simulink model "TST_AFS_VD"  (R2016b)
settings: Solver=FixedStepDiscrete  StartTime=0.0  StopTime=simTime  FixedStep=sampleTime  RelTol=1e-3
values from neighbouring files (symbols this model uses):
  testCase = 1    [initTST_AFS_VD_001.m]    (also in initTST_AFS_VD_002.m = 2)
libraries: simulink x15, UnitTest_Lib x12
settings Model: Creator=zhengjinyan  LastModifiedBy=zhengjinyan
settings DebuggingCC: SignalRangeChecking=error
settings ConfigComp: CovEnable=on  RecordCoverage=on  CovFilter=H:\ZJY\T3_NSE_UT\build\UnitTest\AFS_VD\slcov_output\AFS_VD_covfilter.cvf  CovHTMLOptions=-sRT=0  CovHtmlReporting=on  CovSaveCumulativeToWorkspaceVar=on  CovCumulativeVarName=AFS_VD_covCumulativeData  CovCumulativeReport=on  CovShowResultsExplorer=off  CovModelRefEnable=on

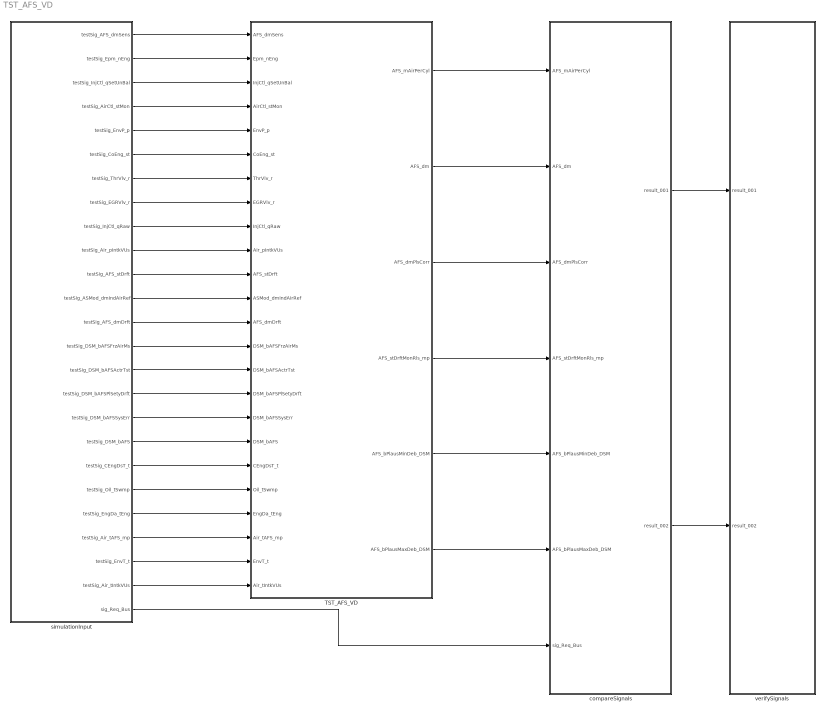
== system TST_AFS_VD ==
  TST_AFS_VD : Subsystem
  compareSignals : Subsystem
  simulationInput : Subsystem
  verifySignals : Subsystem
  wires:
  simulationInput/1(testSig_AFS_dmSens) -> TST_AFS_VD/1(AFS_dmSens)
  simulationInput/2(testSig_Epm_nEng) -> TST_AFS_VD/2(Epm_nEng)
  simulationInput/3(testSig_InjCtl_qSetUnBal) -> TST_AFS_VD/3(InjCtl_qSetUnBal)
  simulationInput/4(testSig_AirCtl_stMon) -> TST_AFS_VD/4(AirCtl_stMon)
  simulationInput/5(testSig_EnvP_p) -> TST_AFS_VD/5(EnvP_p)
  simulationInput/6(testSig_CoEng_st) -> TST_AFS_VD/6(CoEng_st)
  simulationInput/7(testSig_ThrVlv_r) -> TST_AFS_VD/7(ThrVlv_r)
  simulationInput/8(testSig_EGRVlv_r) -> TST_AFS_VD/8(EGRVlv_r)
  simulationInput/9(testSig_InjCtl_qRaw) -> TST_AFS_VD/9(InjCtl_qRaw)
  simulationInput/10(testSig_Air_pIntkVUs) -> TST_AFS_VD/10(Air_pIntkVUs)
  simulationInput/11(testSig_AFS_stDrft) -> TST_AFS_VD/11(AFS_stDrft)
  simulationInput/12(testSig_ASMod_dmIndAirRef) -> TST_AFS_VD/12(ASMod_dmIndAirRef)
  simulationInput/13(testSig_AFS_dmDrft) -> TST_AFS_VD/13(AFS_dmDrft)
  simulationInput/14(testSig_DSM_bAFSFrzAirMs) -> TST_AFS_VD/14(DSM_bAFSFrzAirMs)
  simulationInput/15(testSig_DSM_bAFSActrTst) -> TST_AFS_VD/15(DSM_bAFSActrTst)
  simulationInput/16(testSig_DSM_bAFSPlSetyDrft) -> TST_AFS_VD/16(DSM_bAFSPlSetyDrft)
  simulationInput/17(testSig_DSM_bAFSSysErr) -> TST_AFS_VD/17(DSM_bAFSSysErr)
  simulationInput/18(testSig_DSM_bAFS) -> TST_AFS_VD/18(DSM_bAFS)
  simulationInput/19(testSig_CEngDsT_t) -> TST_AFS_VD/19(CEngDsT_t)
  simulationInput/20(testSig_Oil_tSwmp) -> TST_AFS_VD/20(Oil_tSwmp)
  simulationInput/21(testSig_EngDa_tEng) -> TST_AFS_VD/21(EngDa_tEng)
  simulationInput/22(testSig_Air_tAFS_mp) -> TST_AFS_VD/22(Air_tAFS_mp)
  simulationInput/23(testSig_EnvT_t) -> TST_AFS_VD/23(EnvT_t)
  simulationInput/24(testSig_Air_tIntkVUs) -> TST_AFS_VD/24(Air_tIntkVUs)
  TST_AFS_VD/1(AFS_mAirPerCyl) -> compareSignals/1(AFS_mAirPerCyl)
  TST_AFS_VD/2(AFS_dm) -> compareSignals/2(AFS_dm)
  TST_AFS_VD/3(AFS_dmPlsCorr) -> compareSignals/3(AFS_dmPlsCorr)
  TST_AFS_VD/4(AFS_stDrftMonRls_mp) -> compareSignals/4(AFS_stDrftMonRls_mp)
  TST_AFS_VD/5(AFS_bPlausMinDeb_DSM) -> compareSignals/5(AFS_bPlausMinDeb_DSM)
  TST_AFS_VD/6(AFS_bPlausMaxDeb_DSM) -> compareSignals/6(AFS_bPlausMaxDeb_DSM)
  simulationInput/25(sig_Req_Bus) -> compareSignals/7(sig_Req_Bus)
  compareSignals/1(result_001) -> verifySignals/1(result_001)
  compareSignals/2(result_002) -> verifySignals/2(result_002)

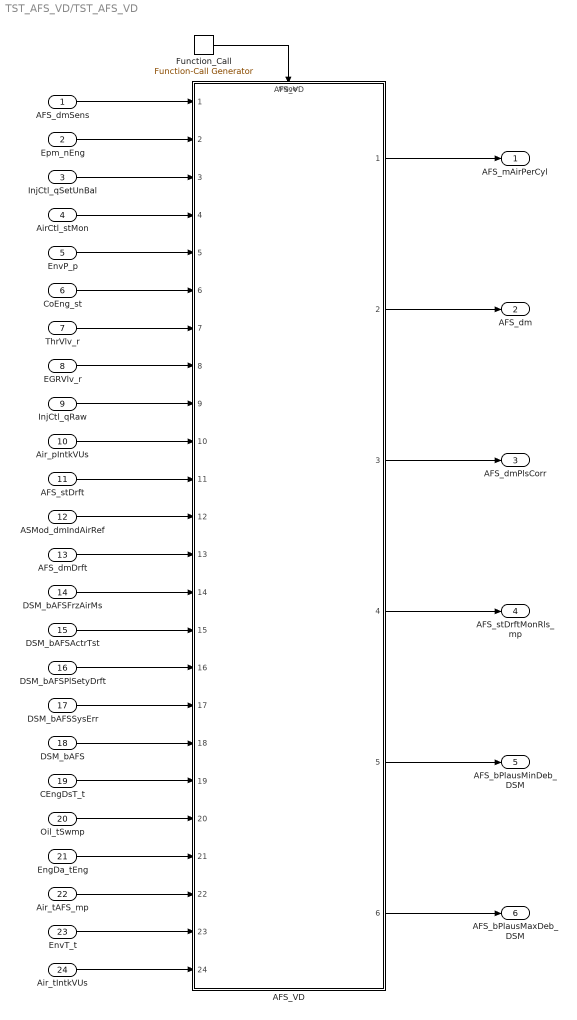
== system TST_AFS_VD/TST_AFS_VD ==
  AFS_dmSens : Inport
  Epm_nEng : Inport  Port=2
  InjCtl_qSetUnBal : Inport  Port=3
  AirCtl_stMon : Inport  Port=4
  EnvP_p : Inport  Port=5
  CoEng_st : Inport  Port=6
  ThrVlv_r : Inport  Port=7
  EGRVlv_r : Inport  Port=8
  InjCtl_qRaw : Inport  Port=9
  Air_pIntkVUs : Inport  Port=10
  AFS_stDrft : Inport  Port=11
  ASMod_dmIndAirRef : Inport  Port=12
  AFS_dmDrft : Inport  Port=13
  DSM_bAFSFrzAirMs : Inport  Port=14
  DSM_bAFSActrTst : Inport  Port=15
  DSM_bAFSPlSetyDrft : Inport  Port=16
  DSM_bAFSSysErr : Inport  Port=17
  DSM_bAFS : Inport  Port=18
  CEngDsT_t : Inport  Port=19
  Oil_tSwmp : Inport  Port=20
  EngDa_tEng : Inport  Port=21
  Air_tAFS_mp : Inport  Port=22
  EnvT_t : Inport  Port=23
  Air_tIntkVUs : Inport  Port=24
  AFS_VD : ModelReference  ModelNameDialog=AFS_VD  SimulationMode=Normal  ModelReferenceVersion=1.64  TriggerPortName=function  TriggerPortTriggerType=function-call  TriggerPortStatesWhenEnabling=held
  Function_Call : simulink/Ports & Subsystems/Function-Call Generator  sample_time=sampleTime  numberOfIterations=1
  AFS_mAirPerCyl : Outport
  AFS_dm : Outport  Port=2
  AFS_dmPlsCorr : Outport  Port=3
  AFS_stDrftMonRls_mp : Outport  Port=4
  AFS_bPlausMinDeb_DSM : Outport  Port=5
  AFS_bPlausMaxDeb_DSM : Outport  Port=6
  wires:
  Function_Call/1 -> AFS_VD/Trigger
  AFS_dmSens/1 -> AFS_VD/1
  Epm_nEng/1 -> AFS_VD/2
  InjCtl_qSetUnBal/1 -> AFS_VD/3
  AirCtl_stMon/1 -> AFS_VD/4
  EnvP_p/1 -> AFS_VD/5
  CoEng_st/1 -> AFS_VD/6
  ThrVlv_r/1 -> AFS_VD/7
  EGRVlv_r/1 -> AFS_VD/8
  InjCtl_qRaw/1 -> AFS_VD/9
  Air_pIntkVUs/1 -> AFS_VD/10
  AFS_stDrft/1 -> AFS_VD/11
  ASMod_dmIndAirRef/1 -> AFS_VD/12
  AFS_dmDrft/1 -> AFS_VD/13
  DSM_bAFSFrzAirMs/1 -> AFS_VD/14
  DSM_bAFSActrTst/1 -> AFS_VD/15
  DSM_bAFSPlSetyDrft/1 -> AFS_VD/16
  DSM_bAFSSysErr/1 -> AFS_VD/17
  DSM_bAFS/1 -> AFS_VD/18
  CEngDsT_t/1 -> AFS_VD/19
  Oil_tSwmp/1 -> AFS_VD/20
  EngDa_tEng/1 -> AFS_VD/21
  Air_tAFS_mp/1 -> AFS_VD/22
  EnvT_t/1 -> AFS_VD/23
  Air_tIntkVUs/1 -> AFS_VD/24
  AFS_VD/1 -> AFS_mAirPerCyl/1
  AFS_VD/2 -> AFS_dm/1
  AFS_VD/3 -> AFS_dmPlsCorr/1
  AFS_VD/4 -> AFS_stDrftMonRls_mp/1
  AFS_VD/5 -> AFS_bPlausMinDeb_DSM/1
  AFS_VD/6 -> AFS_bPlausMaxDeb_DSM/1

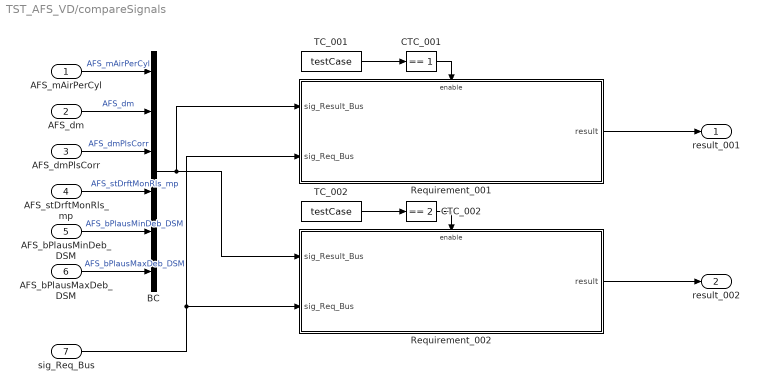
== system TST_AFS_VD/compareSignals ==
  AFS_mAirPerCyl : Inport
  AFS_dm : Inport  Port=2
  AFS_dmPlsCorr : Inport  Port=3
  AFS_stDrftMonRls_mp : Inport  Port=4
  AFS_bPlausMinDeb_DSM : Inport  Port=5
  AFS_bPlausMaxDeb_DSM : Inport  Port=6
  sig_Req_Bus : Inport  Port=7
  BC : BusCreator  Inputs=6
  CTC_001 : simulink/Logic and Bit Operations/Compare To Constant  relop===  const=1  OutDataTypeStr=boolean
  CTC_002 : simulink/Logic and Bit Operations/Compare To Constant  relop===  const=2  OutDataTypeStr=boolean
  Requirement_001 : Subsystem
  Requirement_002 : Subsystem
  TC_001 : Constant  Value=testCase
  TC_002 : Constant  Value=testCase
  result_001 : Outport
  result_002 : Outport  Port=2
  wires:
  AFS_mAirPerCyl/1 -> BC/1  "AFS_mAirPerCyl"
  AFS_dm/1 -> BC/2  "AFS_dm"
  AFS_dmPlsCorr/1 -> BC/3  "AFS_dmPlsCorr"
  AFS_stDrftMonRls_mp/1 -> BC/4  "AFS_stDrftMonRls_mp"
  AFS_bPlausMinDeb_DSM/1 -> BC/5  "AFS_bPlausMinDeb_DSM"
  AFS_bPlausMaxDeb_DSM/1 -> BC/6  "AFS_bPlausMaxDeb_DSM"
  TC_001/1 -> CTC_001/1
  CTC_001/1 -> Requirement_001/Enable
  sig_Req_Bus/1 -> Requirement_001/2(sig_Req_Bus), Requirement_002/2(sig_Req_Bus)
  BC/1 -> Requirement_001/1(sig_Result_Bus), Requirement_002/1(sig_Result_Bus)
  Requirement_001/1(result) -> result_001/1
  TC_002/1 -> CTC_002/1
  CTC_002/1 -> Requirement_002/Enable
  Requirement_002/1(result) -> result_002/1

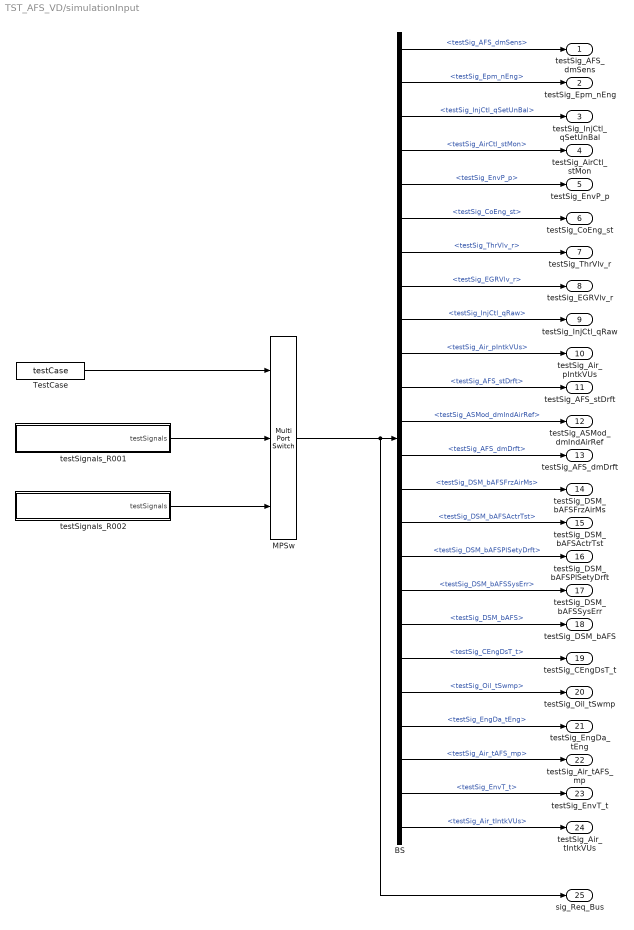
== system TST_AFS_VD/simulationInput ==
  BS : BusSelector  OutputSignals=testSig_AFS_dmSens,testSig_Epm_nEng,testSig_InjCtl_qSetUnBal,testSig_AirCtl_stMon,testSig_EnvP_p,testSig_CoEng_st,testSig_ThrVlv_r,testSig_EGRVlv_r,testSig_InjCtl_qRaw,testSig_Air_pIntkVUs,testSig_AFS_stDrft,testSig_ASMod_dmIndAirRef,testSig_AFS_dmDrft,testSig_DSM_bAFSFrzAirMs,testSig_DSM_bAFSActrTst,testSig_DSM_bAFSPlSetyDrft,testSig_DSM_bAFSSysErr,testSig_DSM_bAFS,testSig_CEngDsT_t,testSig_Oil_tSwmp,testSig_EngDa_tEng,testSig_Air_tAFS_mp,testSig_EnvT_t,testSig_Air_tIntkVUs
  MPSw : MultiPortSwitch  Inputs=2  SaturateOnIntegerOverflow=on  InputSameDT=on
  TestCase : Constant  Value=testCase
  testSignals_R001 : Subsystem
  testSignals_R002 : Subsystem
  testSig_AFS_dmSens : Outport
  testSig_Epm_nEng : Outport  Port=2
  testSig_InjCtl_qSetUnBal : Outport  Port=3
  testSig_AirCtl_stMon : Outport  Port=4
  testSig_EnvP_p : Outport  Port=5
  testSig_CoEng_st : Outport  Port=6
  testSig_ThrVlv_r : Outport  Port=7
  testSig_EGRVlv_r : Outport  Port=8
  testSig_InjCtl_qRaw : Outport  Port=9
  testSig_Air_pIntkVUs : Outport  Port=10
  testSig_AFS_stDrft : Outport  Port=11
  testSig_ASMod_dmIndAirRef : Outport  Port=12
  testSig_AFS_dmDrft : Outport  Port=13
  testSig_DSM_bAFSFrzAirMs : Outport  Port=14
  testSig_DSM_bAFSActrTst : Outport  Port=15
  testSig_DSM_bAFSPlSetyDrft : Outport  Port=16
  testSig_DSM_bAFSSysErr : Outport  Port=17
  testSig_DSM_bAFS : Outport  Port=18
  testSig_CEngDsT_t : Outport  Port=19
  testSig_Oil_tSwmp : Outport  Port=20
  testSig_EngDa_tEng : Outport  Port=21
  testSig_Air_tAFS_mp : Outport  Port=22
  testSig_EnvT_t : Outport  Port=23
  testSig_Air_tIntkVUs : Outport  Port=24
  sig_Req_Bus : Outport  Port=25
  wires:
  BS/1 -> testSig_AFS_dmSens/1  "<testSig_AFS_dmSens>"
  BS/2 -> testSig_Epm_nEng/1  "<testSig_Epm_nEng>"
  BS/3 -> testSig_InjCtl_qSetUnBal/1  "<testSig_InjCtl_qSetUnBal>"
  BS/4 -> testSig_AirCtl_stMon/1  "<testSig_AirCtl_stMon>"
  BS/5 -> testSig_EnvP_p/1  "<testSig_EnvP_p>"
  BS/6 -> testSig_CoEng_st/1  "<testSig_CoEng_st>"
  BS/7 -> testSig_ThrVlv_r/1  "<testSig_ThrVlv_r>"
  BS/8 -> testSig_EGRVlv_r/1  "<testSig_EGRVlv_r>"
  BS/9 -> testSig_InjCtl_qRaw/1  "<testSig_InjCtl_qRaw>"
  BS/10 -> testSig_Air_pIntkVUs/1  "<testSig_Air_pIntkVUs>"
  BS/11 -> testSig_AFS_stDrft/1  "<testSig_AFS_stDrft>"
  BS/12 -> testSig_ASMod_dmIndAirRef/1  "<testSig_ASMod_dmIndAirRef>"
  BS/13 -> testSig_AFS_dmDrft/1  "<testSig_AFS_dmDrft>"
  BS/14 -> testSig_DSM_bAFSFrzAirMs/1  "<testSig_DSM_bAFSFrzAirMs>"
  BS/15 -> testSig_DSM_bAFSActrTst/1  "<testSig_DSM_bAFSActrTst>"
  BS/16 -> testSig_DSM_bAFSPlSetyDrft/1  "<testSig_DSM_bAFSPlSetyDrft>"
  BS/17 -> testSig_DSM_bAFSSysErr/1  "<testSig_DSM_bAFSSysErr>"
  BS/18 -> testSig_DSM_bAFS/1  "<testSig_DSM_bAFS>"
  BS/19 -> testSig_CEngDsT_t/1  "<testSig_CEngDsT_t>"
  BS/20 -> testSig_Oil_tSwmp/1  "<testSig_Oil_tSwmp>"
  BS/21 -> testSig_EngDa_tEng/1  "<testSig_EngDa_tEng>"
  BS/22 -> testSig_Air_tAFS_mp/1  "<testSig_Air_tAFS_mp>"
  BS/23 -> testSig_EnvT_t/1  "<testSig_EnvT_t>"
  BS/24 -> testSig_Air_tIntkVUs/1  "<testSig_Air_tIntkVUs>"
  MPSw/1 -> BS/1, sig_Req_Bus/1
  TestCase/1 -> MPSw/1
  testSignals_R001/1(testSignals) -> MPSw/2
  testSignals_R002/1(testSignals) -> MPSw/3

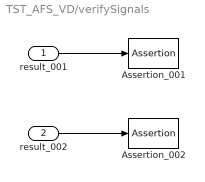
== system TST_AFS_VD/verifySignals ==
  result_001 : Inport
  result_002 : Inport  Port=2
  Assertion_001 : Assertion  Enabled=off
  Assertion_002 : Assertion  Enabled=off
  wires:
  result_001/1 -> Assertion_001/1
  result_002/1 -> Assertion_002/1

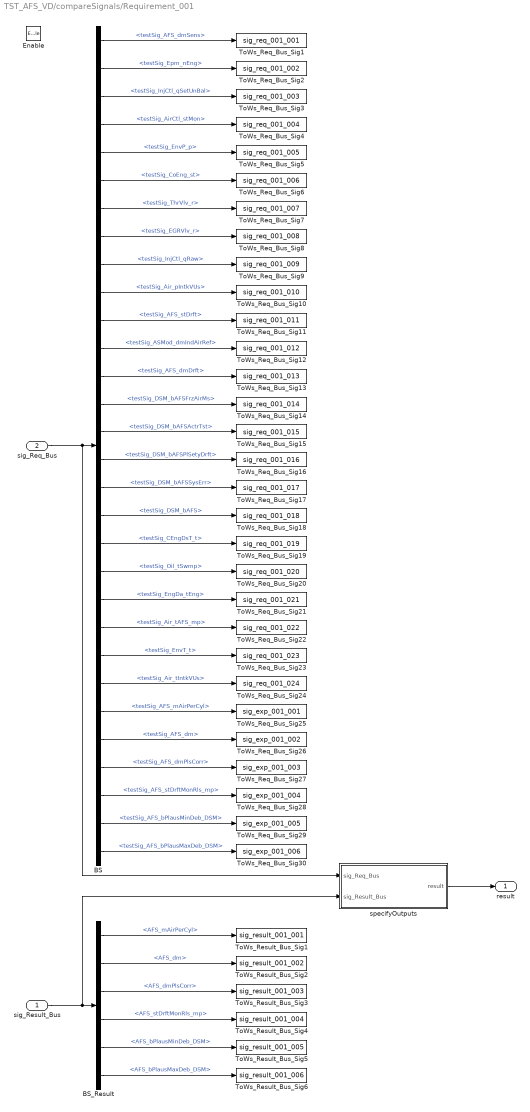
== system TST_AFS_VD/compareSignals/Requirement_001 ==
  sig_Result_Bus : Inport
  sig_Req_Bus : Inport  Port=2
  Enable : EnablePort
  BS : BusSelector  OutputSignals=testSig_AFS_dmSens,testSig_Epm_nEng,testSig_InjCtl_qSetUnBal,testSig_AirCtl_stMon,testSig_EnvP_p,testSig_CoEng_st,testSig_ThrVlv_r,testSig_EGRVlv_r,testSig_InjCtl_qRaw,testSig_Air_pIntkVUs,testSig_AFS_stDrft,testSig_ASMod_dmIndAirRef,testSig_AFS_dmDrft,testSig_DSM_bAFSFrzAirMs,testSig_DSM_bAFSActrTst,testSig_DSM_bAFSPlSetyDrft,testSig_DSM_bAFSSysErr,testSig_DSM_bAFS,testSig_CEngDsT_t,testSig_Oil_tSwmp,testSig_EngDa_tEng,testSig_Air_tAFS_mp,testSig_EnvT_t,testSig_Air_tIntkVUs,testSig_AFS_mAirPerCyl,testSig_AFS_dm,testSig_AFS_dmPlsCorr,testSig_AFS_stDrftMonRls_mp,testSig_AFS_bPlausMinDeb_DSM,testSig_AFS_bPlausMaxDeb_DSM
  BS_Result : BusSelector  OutputSignals=AFS_mAirPerCyl,AFS_dm,AFS_dmPlsCorr,AFS_stDrftMonRls_mp,AFS_bPlausMinDeb_DSM,AFS_bPlausMaxDeb_DSM
  ToWs_Req_Bus_Sig1 : ToWorkspace  VariableName=sig_req_001_001  SaveFormat=Structure With Time
  ToWs_Req_Bus_Sig10 : ToWorkspace  VariableName=sig_req_001_010  SaveFormat=Structure With Time
  ToWs_Req_Bus_Sig11 : ToWorkspace  VariableName=sig_req_001_011  SaveFormat=Structure With Time
  ToWs_Req_Bus_Sig12 : ToWorkspace  VariableName=sig_req_001_012  SaveFormat=Structure With Time
  ToWs_Req_Bus_Sig13 : ToWorkspace  VariableName=sig_req_001_013  SaveFormat=Structure With Time
  ToWs_Req_Bus_Sig14 : ToWorkspace  VariableName=sig_req_001_014  SaveFormat=Structure With Time
  ToWs_Req_Bus_Sig15 : ToWorkspace  VariableName=sig_req_001_015  SaveFormat=Structure With Time
  ToWs_Req_Bus_Sig16 : ToWorkspace  VariableName=sig_req_001_016  SaveFormat=Structure With Time
  ToWs_Req_Bus_Sig17 : ToWorkspace  VariableName=sig_req_001_017  SaveFormat=Structure With Time
  ToWs_Req_Bus_Sig18 : ToWorkspace  VariableName=sig_req_001_018  SaveFormat=Structure With Time
  ToWs_Req_Bus_Sig19 : ToWorkspace  VariableName=sig_req_001_019  SaveFormat=Structure With Time
  ToWs_Req_Bus_Sig2 : ToWorkspace  VariableName=sig_req_001_002  SaveFormat=Structure With Time
  ToWs_Req_Bus_Sig20 : ToWorkspace  VariableName=sig_req_001_020  SaveFormat=Structure With Time
  ToWs_Req_Bus_Sig21 : ToWorkspace  VariableName=sig_req_001_021  SaveFormat=Structure With Time
  ToWs_Req_Bus_Sig22 : ToWorkspace  VariableName=sig_req_001_022  SaveFormat=Structure With Time
  ToWs_Req_Bus_Sig23 : ToWorkspace  VariableName=sig_req_001_023  SaveFormat=Structure With Time
  ToWs_Req_Bus_Sig24 : ToWorkspace  VariableName=sig_req_001_024  SaveFormat=Structure With Time
  ToWs_Req_Bus_Sig25 : ToWorkspace  VariableName=sig_exp_001_001  SaveFormat=Structure With Time
  ToWs_Req_Bus_Sig26 : ToWorkspace  VariableName=sig_exp_001_002  SaveFormat=Structure With Time
  ToWs_Req_Bus_Sig27 : ToWorkspace  VariableName=sig_exp_001_003  SaveFormat=Structure With Time
  ToWs_Req_Bus_Sig28 : ToWorkspace  VariableName=sig_exp_001_004  SaveFormat=Structure With Time
  ToWs_Req_Bus_Sig29 : ToWorkspace  VariableName=sig_exp_001_005  SaveFormat=Structure With Time
  ToWs_Req_Bus_Sig3 : ToWorkspace  VariableName=sig_req_001_003  SaveFormat=Structure With Time
  ToWs_Req_Bus_Sig30 : ToWorkspace  VariableName=sig_exp_001_006  SaveFormat=Structure With Time
  ToWs_Req_Bus_Sig4 : ToWorkspace  VariableName=sig_req_001_004  SaveFormat=Structure With Time
  ToWs_Req_Bus_Sig5 : ToWorkspace  VariableName=sig_req_001_005  SaveFormat=Structure With Time
  ToWs_Req_Bus_Sig6 : ToWorkspace  VariableName=sig_req_001_006  SaveFormat=Structure With Time
  ToWs_Req_Bus_Sig7 : ToWorkspace  VariableName=sig_req_001_007  SaveFormat=Structure With Time
  ToWs_Req_Bus_Sig8 : ToWorkspace  VariableName=sig_req_001_008  SaveFormat=Structure With Time
  ToWs_Req_Bus_Sig9 : ToWorkspace  VariableName=sig_req_001_009  SaveFormat=Structure With Time
  ToWs_Result_Bus_Sig1 : ToWorkspace  VariableName=sig_result_001_001  SaveFormat=Structure With Time
  ToWs_Result_Bus_Sig2 : ToWorkspace  VariableName=sig_result_001_002  SaveFormat=Structure With Time
  ToWs_Result_Bus_Sig3 : ToWorkspace  VariableName=sig_result_001_003  SaveFormat=Structure With Time
  ToWs_Result_Bus_Sig4 : ToWorkspace  VariableName=sig_result_001_004  SaveFormat=Structure With Time
  ToWs_Result_Bus_Sig5 : ToWorkspace  VariableName=sig_result_001_005  SaveFormat=Structure With Time
  ToWs_Result_Bus_Sig6 : ToWorkspace  VariableName=sig_result_001_006  SaveFormat=Structure With Time
  specifyOutputs : Subsystem
  result : Outport
  wires:
  sig_Req_Bus/1 -> BS/1, specifyOutputs/1(sig_Req_Bus)
  BS/1 -> ToWs_Req_Bus_Sig1/1  "<testSig_AFS_dmSens>"
  BS/2 -> ToWs_Req_Bus_Sig2/1  "<testSig_Epm_nEng>"
  BS/3 -> ToWs_Req_Bus_Sig3/1  "<testSig_InjCtl_qSetUnBal>"
  BS/4 -> ToWs_Req_Bus_Sig4/1  "<testSig_AirCtl_stMon>"
  BS/5 -> ToWs_Req_Bus_Sig5/1  "<testSig_EnvP_p>"
  BS/6 -> ToWs_Req_Bus_Sig6/1  "<testSig_CoEng_st>"
  BS/7 -> ToWs_Req_Bus_Sig7/1  "<testSig_ThrVlv_r>"
  BS/8 -> ToWs_Req_Bus_Sig8/1  "<testSig_EGRVlv_r>"
  BS/9 -> ToWs_Req_Bus_Sig9/1  "<testSig_InjCtl_qRaw>"
  BS/10 -> ToWs_Req_Bus_Sig10/1  "<testSig_Air_pIntkVUs>"
  BS/11 -> ToWs_Req_Bus_Sig11/1  "<testSig_AFS_stDrft>"
  BS/12 -> ToWs_Req_Bus_Sig12/1  "<testSig_ASMod_dmIndAirRef>"
  BS/13 -> ToWs_Req_Bus_Sig13/1  "<testSig_AFS_dmDrft>"
  BS/14 -> ToWs_Req_Bus_Sig14/1  "<testSig_DSM_bAFSFrzAirMs>"
  BS/15 -> ToWs_Req_Bus_Sig15/1  "<testSig_DSM_bAFSActrTst>"
  BS/16 -> ToWs_Req_Bus_Sig16/1  "<testSig_DSM_bAFSPlSetyDrft>"
  BS/17 -> ToWs_Req_Bus_Sig17/1  "<testSig_DSM_bAFSSysErr>"
  BS/18 -> ToWs_Req_Bus_Sig18/1  "<testSig_DSM_bAFS>"
  BS/19 -> ToWs_Req_Bus_Sig19/1  "<testSig_CEngDsT_t>"
  BS/20 -> ToWs_Req_Bus_Sig20/1  "<testSig_Oil_tSwmp>"
  BS/21 -> ToWs_Req_Bus_Sig21/1  "<testSig_EngDa_tEng>"
  BS/22 -> ToWs_Req_Bus_Sig22/1  "<testSig_Air_tAFS_mp>"
  BS/23 -> ToWs_Req_Bus_Sig23/1  "<testSig_EnvT_t>"
  BS/24 -> ToWs_Req_Bus_Sig24/1  "<testSig_Air_tIntkVUs>"
  BS/25 -> ToWs_Req_Bus_Sig25/1  "<testSig_AFS_mAirPerCyl>"
  BS/26 -> ToWs_Req_Bus_Sig26/1  "<testSig_AFS_dm>"
  BS/27 -> ToWs_Req_Bus_Sig27/1  "<testSig_AFS_dmPlsCorr>"
  BS/28 -> ToWs_Req_Bus_Sig28/1  "<testSig_AFS_stDrftMonRls_mp>"
  BS/29 -> ToWs_Req_Bus_Sig29/1  "<testSig_AFS_bPlausMinDeb_DSM>"
  BS/30 -> ToWs_Req_Bus_Sig30/1  "<testSig_AFS_bPlausMaxDeb_DSM>"
  sig_Result_Bus/1 -> BS_Result/1, specifyOutputs/2(sig_Result_Bus)
  BS_Result/1 -> ToWs_Result_Bus_Sig1/1  "<AFS_mAirPerCyl>"
  BS_Result/2 -> ToWs_Result_Bus_Sig2/1  "<AFS_dm>"
  BS_Result/3 -> ToWs_Result_Bus_Sig3/1  "<AFS_dmPlsCorr>"
  BS_Result/4 -> ToWs_Result_Bus_Sig4/1  "<AFS_stDrftMonRls_mp>"
  BS_Result/5 -> ToWs_Result_Bus_Sig5/1  "<AFS_bPlausMinDeb_DSM>"
  BS_Result/6 -> ToWs_Result_Bus_Sig6/1  "<AFS_bPlausMaxDeb_DSM>"
  specifyOutputs/1(result) -> result/1

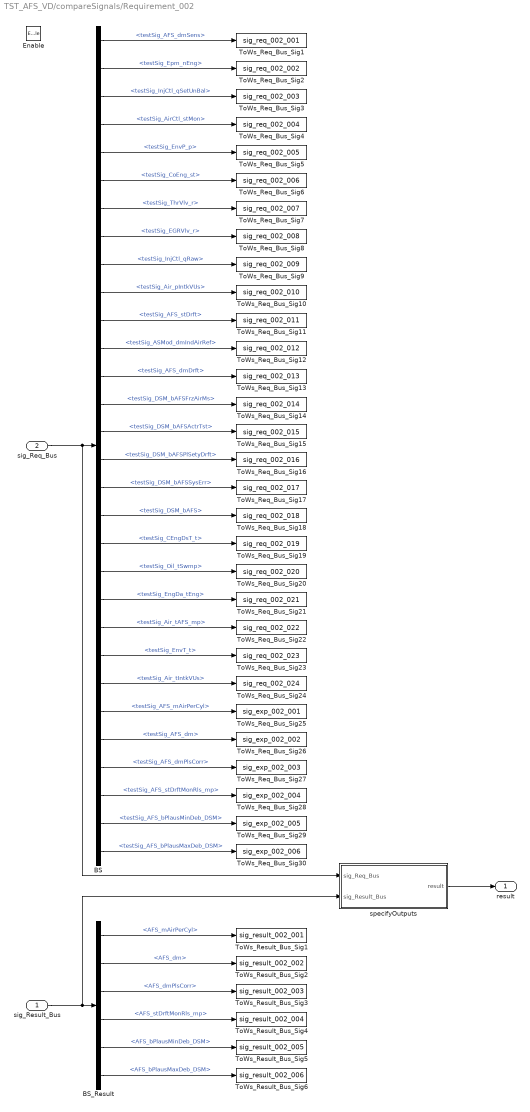
== system TST_AFS_VD/compareSignals/Requirement_002 ==
  sig_Result_Bus : Inport
  sig_Req_Bus : Inport  Port=2
  Enable : EnablePort
  BS : BusSelector  OutputSignals=testSig_AFS_dmSens,testSig_Epm_nEng,testSig_InjCtl_qSetUnBal,testSig_AirCtl_stMon,testSig_EnvP_p,testSig_CoEng_st,testSig_ThrVlv_r,testSig_EGRVlv_r,testSig_InjCtl_qRaw,testSig_Air_pIntkVUs,testSig_AFS_stDrft,testSig_ASMod_dmIndAirRef,testSig_AFS_dmDrft,testSig_DSM_bAFSFrzAirMs,testSig_DSM_bAFSActrTst,testSig_DSM_bAFSPlSetyDrft,testSig_DSM_bAFSSysErr,testSig_DSM_bAFS,testSig_CEngDsT_t,testSig_Oil_tSwmp,testSig_EngDa_tEng,testSig_Air_tAFS_mp,testSig_EnvT_t,testSig_Air_tIntkVUs,testSig_AFS_mAirPerCyl,testSig_AFS_dm,testSig_AFS_dmPlsCorr,testSig_AFS_stDrftMonRls_mp,testSig_AFS_bPlausMinDeb_DSM,testSig_AFS_bPlausMaxDeb_DSM
  BS_Result : BusSelector  OutputSignals=AFS_mAirPerCyl,AFS_dm,AFS_dmPlsCorr,AFS_stDrftMonRls_mp,AFS_bPlausMinDeb_DSM,AFS_bPlausMaxDeb_DSM
  ToWs_Req_Bus_Sig1 : ToWorkspace  VariableName=sig_req_002_001  SaveFormat=Structure With Time
  ToWs_Req_Bus_Sig10 : ToWorkspace  VariableName=sig_req_002_010  SaveFormat=Structure With Time
  ToWs_Req_Bus_Sig11 : ToWorkspace  VariableName=sig_req_002_011  SaveFormat=Structure With Time
  ToWs_Req_Bus_Sig12 : ToWorkspace  VariableName=sig_req_002_012  SaveFormat=Structure With Time
  ToWs_Req_Bus_Sig13 : ToWorkspace  VariableName=sig_req_002_013  SaveFormat=Structure With Time
  ToWs_Req_Bus_Sig14 : ToWorkspace  VariableName=sig_req_002_014  SaveFormat=Structure With Time
  ToWs_Req_Bus_Sig15 : ToWorkspace  VariableName=sig_req_002_015  SaveFormat=Structure With Time
  ToWs_Req_Bus_Sig16 : ToWorkspace  VariableName=sig_req_002_016  SaveFormat=Structure With Time
  ToWs_Req_Bus_Sig17 : ToWorkspace  VariableName=sig_req_002_017  SaveFormat=Structure With Time
  ToWs_Req_Bus_Sig18 : ToWorkspace  VariableName=sig_req_002_018  SaveFormat=Structure With Time
  ToWs_Req_Bus_Sig19 : ToWorkspace  VariableName=sig_req_002_019  SaveFormat=Structure With Time
  ToWs_Req_Bus_Sig2 : ToWorkspace  VariableName=sig_req_002_002  SaveFormat=Structure With Time
  ToWs_Req_Bus_Sig20 : ToWorkspace  VariableName=sig_req_002_020  SaveFormat=Structure With Time
  ToWs_Req_Bus_Sig21 : ToWorkspace  VariableName=sig_req_002_021  SaveFormat=Structure With Time
  ToWs_Req_Bus_Sig22 : ToWorkspace  VariableName=sig_req_002_022  SaveFormat=Structure With Time
  ToWs_Req_Bus_Sig23 : ToWorkspace  VariableName=sig_req_002_023  SaveFormat=Structure With Time
  ToWs_Req_Bus_Sig24 : ToWorkspace  VariableName=sig_req_002_024  SaveFormat=Structure With Time
  ToWs_Req_Bus_Sig25 : ToWorkspace  VariableName=sig_exp_002_001  SaveFormat=Structure With Time
  ToWs_Req_Bus_Sig26 : ToWorkspace  VariableName=sig_exp_002_002  SaveFormat=Structure With Time
  ToWs_Req_Bus_Sig27 : ToWorkspace  VariableName=sig_exp_002_003  SaveFormat=Structure With Time
  ToWs_Req_Bus_Sig28 : ToWorkspace  VariableName=sig_exp_002_004  SaveFormat=Structure With Time
  ToWs_Req_Bus_Sig29 : ToWorkspace  VariableName=sig_exp_002_005  SaveFormat=Structure With Time
  ToWs_Req_Bus_Sig3 : ToWorkspace  VariableName=sig_req_002_003  SaveFormat=Structure With Time
  ToWs_Req_Bus_Sig30 : ToWorkspace  VariableName=sig_exp_002_006  SaveFormat=Structure With Time
  ToWs_Req_Bus_Sig4 : ToWorkspace  VariableName=sig_req_002_004  SaveFormat=Structure With Time
  ToWs_Req_Bus_Sig5 : ToWorkspace  VariableName=sig_req_002_005  SaveFormat=Structure With Time
  ToWs_Req_Bus_Sig6 : ToWorkspace  VariableName=sig_req_002_006  SaveFormat=Structure With Time
  ToWs_Req_Bus_Sig7 : ToWorkspace  VariableName=sig_req_002_007  SaveFormat=Structure With Time
  ToWs_Req_Bus_Sig8 : ToWorkspace  VariableName=sig_req_002_008  SaveFormat=Structure With Time
  ToWs_Req_Bus_Sig9 : ToWorkspace  VariableName=sig_req_002_009  SaveFormat=Structure With Time
  ToWs_Result_Bus_Sig1 : ToWorkspace  VariableName=sig_result_002_001  SaveFormat=Structure With Time
  ToWs_Result_Bus_Sig2 : ToWorkspace  VariableName=sig_result_002_002  SaveFormat=Structure With Time
  ToWs_Result_Bus_Sig3 : ToWorkspace  VariableName=sig_result_002_003  SaveFormat=Structure With Time
  ToWs_Result_Bus_Sig4 : ToWorkspace  VariableName=sig_result_002_004  SaveFormat=Structure With Time
  ToWs_Result_Bus_Sig5 : ToWorkspace  VariableName=sig_result_002_005  SaveFormat=Structure With Time
  ToWs_Result_Bus_Sig6 : ToWorkspace  VariableName=sig_result_002_006  SaveFormat=Structure With Time
  specifyOutputs : Subsystem
  result : Outport
  wires:
  sig_Req_Bus/1 -> BS/1, specifyOutputs/1(sig_Req_Bus)
  BS/1 -> ToWs_Req_Bus_Sig1/1  "<testSig_AFS_dmSens>"
  BS/2 -> ToWs_Req_Bus_Sig2/1  "<testSig_Epm_nEng>"
  BS/3 -> ToWs_Req_Bus_Sig3/1  "<testSig_InjCtl_qSetUnBal>"
  BS/4 -> ToWs_Req_Bus_Sig4/1  "<testSig_AirCtl_stMon>"
  BS/5 -> ToWs_Req_Bus_Sig5/1  "<testSig_EnvP_p>"
  BS/6 -> ToWs_Req_Bus_Sig6/1  "<testSig_CoEng_st>"
  BS/7 -> ToWs_Req_Bus_Sig7/1  "<testSig_ThrVlv_r>"
  BS/8 -> ToWs_Req_Bus_Sig8/1  "<testSig_EGRVlv_r>"
  BS/9 -> ToWs_Req_Bus_Sig9/1  "<testSig_InjCtl_qRaw>"
  BS/10 -> ToWs_Req_Bus_Sig10/1  "<testSig_Air_pIntkVUs>"
  BS/11 -> ToWs_Req_Bus_Sig11/1  "<testSig_AFS_stDrft>"
  BS/12 -> ToWs_Req_Bus_Sig12/1  "<testSig_ASMod_dmIndAirRef>"
  BS/13 -> ToWs_Req_Bus_Sig13/1  "<testSig_AFS_dmDrft>"
  BS/14 -> ToWs_Req_Bus_Sig14/1  "<testSig_DSM_bAFSFrzAirMs>"
  BS/15 -> ToWs_Req_Bus_Sig15/1  "<testSig_DSM_bAFSActrTst>"
  BS/16 -> ToWs_Req_Bus_Sig16/1  "<testSig_DSM_bAFSPlSetyDrft>"
  BS/17 -> ToWs_Req_Bus_Sig17/1  "<testSig_DSM_bAFSSysErr>"
  BS/18 -> ToWs_Req_Bus_Sig18/1  "<testSig_DSM_bAFS>"
  BS/19 -> ToWs_Req_Bus_Sig19/1  "<testSig_CEngDsT_t>"
  BS/20 -> ToWs_Req_Bus_Sig20/1  "<testSig_Oil_tSwmp>"
  BS/21 -> ToWs_Req_Bus_Sig21/1  "<testSig_EngDa_tEng>"
  BS/22 -> ToWs_Req_Bus_Sig22/1  "<testSig_Air_tAFS_mp>"
  BS/23 -> ToWs_Req_Bus_Sig23/1  "<testSig_EnvT_t>"
  BS/24 -> ToWs_Req_Bus_Sig24/1  "<testSig_Air_tIntkVUs>"
  BS/25 -> ToWs_Req_Bus_Sig25/1  "<testSig_AFS_mAirPerCyl>"
  BS/26 -> ToWs_Req_Bus_Sig26/1  "<testSig_AFS_dm>"
  BS/27 -> ToWs_Req_Bus_Sig27/1  "<testSig_AFS_dmPlsCorr>"
  BS/28 -> ToWs_Req_Bus_Sig28/1  "<testSig_AFS_stDrftMonRls_mp>"
  BS/29 -> ToWs_Req_Bus_Sig29/1  "<testSig_AFS_bPlausMinDeb_DSM>"
  BS/30 -> ToWs_Req_Bus_Sig30/1  "<testSig_AFS_bPlausMaxDeb_DSM>"
  sig_Result_Bus/1 -> BS_Result/1, specifyOutputs/2(sig_Result_Bus)
  BS_Result/1 -> ToWs_Result_Bus_Sig1/1  "<AFS_mAirPerCyl>"
  BS_Result/2 -> ToWs_Result_Bus_Sig2/1  "<AFS_dm>"
  BS_Result/3 -> ToWs_Result_Bus_Sig3/1  "<AFS_dmPlsCorr>"
  BS_Result/4 -> ToWs_Result_Bus_Sig4/1  "<AFS_stDrftMonRls_mp>"
  BS_Result/5 -> ToWs_Result_Bus_Sig5/1  "<AFS_bPlausMinDeb_DSM>"
  BS_Result/6 -> ToWs_Result_Bus_Sig6/1  "<AFS_bPlausMaxDeb_DSM>"
  specifyOutputs/1(result) -> result/1

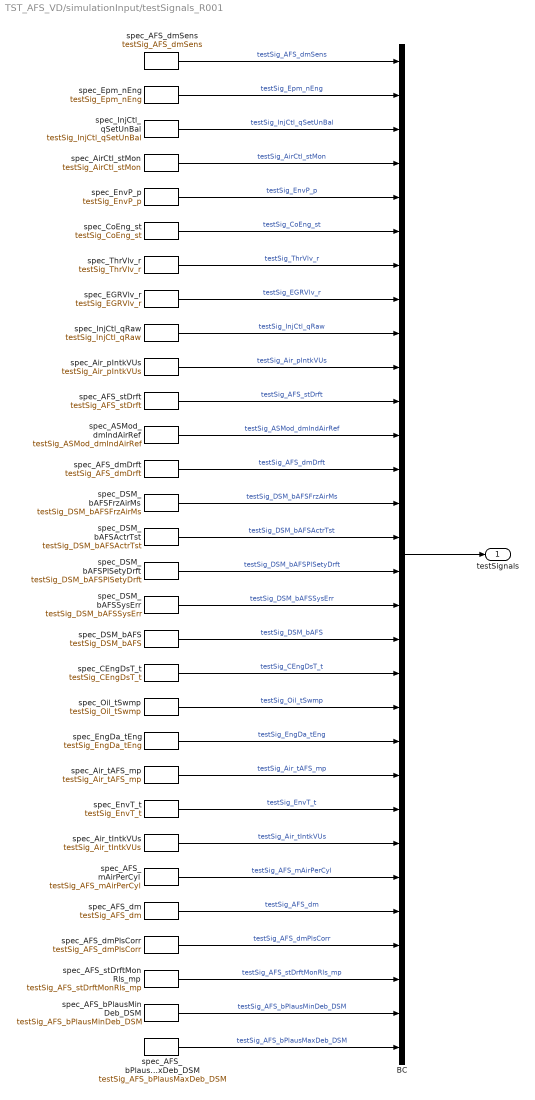
== system TST_AFS_VD/simulationInput/testSignals_R001 ==
  BC : BusCreator  Inputs=30
  spec_AFS_bPlausMaxDeb_DSM : FromWorkspace  VariableName=testSig_AFS_bPlausMaxDeb_DSM  Interpolate=off  OutputAfterFinalValue=Holding final value
  spec_AFS_bPlausMinDeb_DSM : FromWorkspace  VariableName=testSig_AFS_bPlausMinDeb_DSM  Interpolate=off  OutputAfterFinalValue=Holding final value
  spec_AFS_dm : FromWorkspace  VariableName=testSig_AFS_dm  Interpolate=off  OutputAfterFinalValue=Holding final value
  spec_AFS_dmDrft : FromWorkspace  VariableName=testSig_AFS_dmDrft  Interpolate=off  OutputAfterFinalValue=Holding final value
  spec_AFS_dmPlsCorr : FromWorkspace  VariableName=testSig_AFS_dmPlsCorr  Interpolate=off  OutputAfterFinalValue=Holding final value
  spec_AFS_dmSens : FromWorkspace  VariableName=testSig_AFS_dmSens  Interpolate=off  OutputAfterFinalValue=Holding final value
  spec_AFS_mAirPerCyl : FromWorkspace  VariableName=testSig_AFS_mAirPerCyl  Interpolate=off  OutputAfterFinalValue=Holding final value
  spec_AFS_stDrft : FromWorkspace  VariableName=testSig_AFS_stDrft  Interpolate=off  OutputAfterFinalValue=Holding final value
  spec_AFS_stDrftMonRls_mp : FromWorkspace  VariableName=testSig_AFS_stDrftMonRls_mp  Interpolate=off  OutputAfterFinalValue=Holding final value
  spec_ASMod_dmIndAirRef : FromWorkspace  VariableName=testSig_ASMod_dmIndAirRef  Interpolate=off  OutputAfterFinalValue=Holding final value
  spec_AirCtl_stMon : FromWorkspace  VariableName=testSig_AirCtl_stMon  Interpolate=off  OutputAfterFinalValue=Holding final value
  spec_Air_pIntkVUs : FromWorkspace  VariableName=testSig_Air_pIntkVUs  Interpolate=off  OutputAfterFinalValue=Holding final value
  spec_Air_tAFS_mp : FromWorkspace  VariableName=testSig_Air_tAFS_mp  Interpolate=off  OutputAfterFinalValue=Holding final value
  spec_Air_tIntkVUs : FromWorkspace  VariableName=testSig_Air_tIntkVUs  Interpolate=off  OutputAfterFinalValue=Holding final value
  spec_CEngDsT_t : FromWorkspace  VariableName=testSig_CEngDsT_t  Interpolate=off  OutputAfterFinalValue=Holding final value
  spec_CoEng_st : FromWorkspace  VariableName=testSig_CoEng_st  Interpolate=off  OutputAfterFinalValue=Holding final value
  spec_DSM_bAFS : FromWorkspace  VariableName=testSig_DSM_bAFS  Interpolate=off  OutputAfterFinalValue=Holding final value
  spec_DSM_bAFSActrTst : FromWorkspace  VariableName=testSig_DSM_bAFSActrTst  Interpolate=off  OutputAfterFinalValue=Holding final value
  spec_DSM_bAFSFrzAirMs : FromWorkspace  VariableName=testSig_DSM_bAFSFrzAirMs  Interpolate=off  OutputAfterFinalValue=Holding final value
  spec_DSM_bAFSPlSetyDrft : FromWorkspace  VariableName=testSig_DSM_bAFSPlSetyDrft  Interpolate=off  OutputAfterFinalValue=Holding final value
  spec_DSM_bAFSSysErr : FromWorkspace  VariableName=testSig_DSM_bAFSSysErr  Interpolate=off  OutputAfterFinalValue=Holding final value
  spec_EGRVlv_r : FromWorkspace  VariableName=testSig_EGRVlv_r  Interpolate=off  OutputAfterFinalValue=Holding final value
  spec_EngDa_tEng : FromWorkspace  VariableName=testSig_EngDa_tEng  Interpolate=off  OutputAfterFinalValue=Holding final value
  spec_EnvP_p : FromWorkspace  VariableName=testSig_EnvP_p  Interpolate=off  OutputAfterFinalValue=Holding final value
  spec_EnvT_t : FromWorkspace  VariableName=testSig_EnvT_t  Interpolate=off  OutputAfterFinalValue=Holding final value
  spec_Epm_nEng : FromWorkspace  VariableName=testSig_Epm_nEng  Interpolate=off  OutputAfterFinalValue=Holding final value
  spec_InjCtl_qRaw : FromWorkspace  VariableName=testSig_InjCtl_qRaw  Interpolate=off  OutputAfterFinalValue=Holding final value
  spec_InjCtl_qSetUnBal : FromWorkspace  VariableName=testSig_InjCtl_qSetUnBal  Interpolate=off  OutputAfterFinalValue=Holding final value
  spec_Oil_tSwmp : FromWorkspace  VariableName=testSig_Oil_tSwmp  Interpolate=off  OutputAfterFinalValue=Holding final value
  spec_ThrVlv_r : FromWorkspace  VariableName=testSig_ThrVlv_r  Interpolate=off  OutputAfterFinalValue=Holding final value
  testSignals : Outport
  wires:
  BC/1 -> testSignals/1
  spec_AFS_dmSens/1 -> BC/1  "testSig_AFS_dmSens"
  spec_Epm_nEng/1 -> BC/2  "testSig_Epm_nEng"
  spec_InjCtl_qSetUnBal/1 -> BC/3  "testSig_InjCtl_qSetUnBal"
  spec_AirCtl_stMon/1 -> BC/4  "testSig_AirCtl_stMon"
  spec_EnvP_p/1 -> BC/5  "testSig_EnvP_p"
  spec_CoEng_st/1 -> BC/6  "testSig_CoEng_st"
  spec_ThrVlv_r/1 -> BC/7  "testSig_ThrVlv_r"
  spec_EGRVlv_r/1 -> BC/8  "testSig_EGRVlv_r"
  spec_InjCtl_qRaw/1 -> BC/9  "testSig_InjCtl_qRaw"
  spec_Air_pIntkVUs/1 -> BC/10  "testSig_Air_pIntkVUs"
  spec_AFS_stDrft/1 -> BC/11  "testSig_AFS_stDrft"
  spec_ASMod_dmIndAirRef/1 -> BC/12  "testSig_ASMod_dmIndAirRef"
  spec_AFS_dmDrft/1 -> BC/13  "testSig_AFS_dmDrft"
  spec_DSM_bAFSFrzAirMs/1 -> BC/14  "testSig_DSM_bAFSFrzAirMs"
  spec_DSM_bAFSActrTst/1 -> BC/15  "testSig_DSM_bAFSActrTst"
  spec_DSM_bAFSPlSetyDrft/1 -> BC/16  "testSig_DSM_bAFSPlSetyDrft"
  spec_DSM_bAFSSysErr/1 -> BC/17  "testSig_DSM_bAFSSysErr"
  spec_DSM_bAFS/1 -> BC/18  "testSig_DSM_bAFS"
  spec_CEngDsT_t/1 -> BC/19  "testSig_CEngDsT_t"
  spec_Oil_tSwmp/1 -> BC/20  "testSig_Oil_tSwmp"
  spec_EngDa_tEng/1 -> BC/21  "testSig_EngDa_tEng"
  spec_Air_tAFS_mp/1 -> BC/22  "testSig_Air_tAFS_mp"
  spec_EnvT_t/1 -> BC/23  "testSig_EnvT_t"
  spec_Air_tIntkVUs/1 -> BC/24  "testSig_Air_tIntkVUs"
  spec_AFS_mAirPerCyl/1 -> BC/25  "testSig_AFS_mAirPerCyl"
  spec_AFS_dm/1 -> BC/26  "testSig_AFS_dm"
  spec_AFS_dmPlsCorr/1 -> BC/27  "testSig_AFS_dmPlsCorr"
  spec_AFS_stDrftMonRls_mp/1 -> BC/28  "testSig_AFS_stDrftMonRls_mp"
  spec_AFS_bPlausMinDeb_DSM/1 -> BC/29  "testSig_AFS_bPlausMinDeb_DSM"
  spec_AFS_bPlausMaxDeb_DSM/1 -> BC/30  "testSig_AFS_bPlausMaxDeb_DSM"

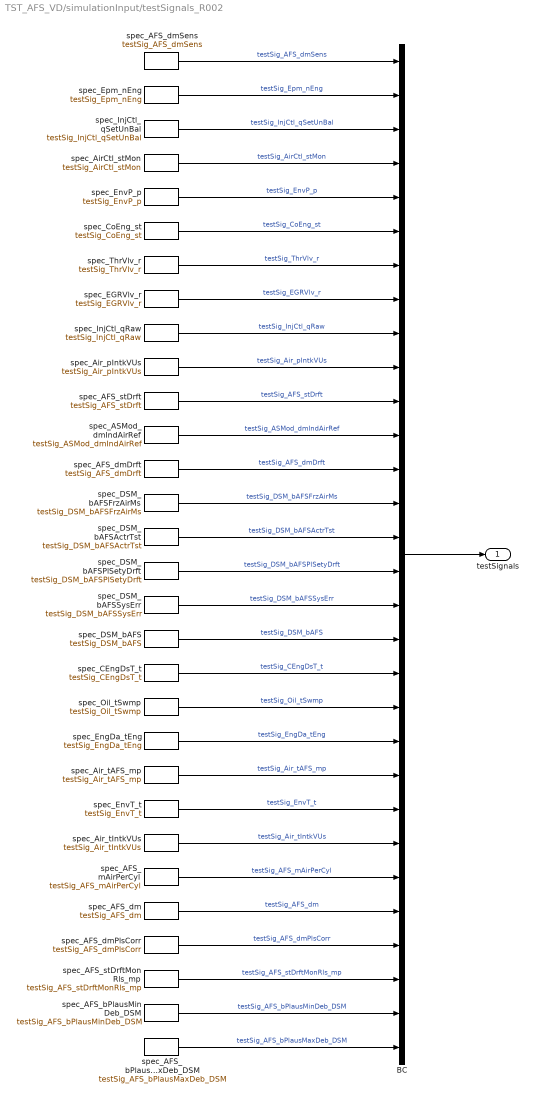
== system TST_AFS_VD/simulationInput/testSignals_R002 ==
  BC : BusCreator  Inputs=30
  spec_AFS_bPlausMaxDeb_DSM : FromWorkspace  VariableName=testSig_AFS_bPlausMaxDeb_DSM  Interpolate=off  OutputAfterFinalValue=Holding final value
  spec_AFS_bPlausMinDeb_DSM : FromWorkspace  VariableName=testSig_AFS_bPlausMinDeb_DSM  Interpolate=off  OutputAfterFinalValue=Holding final value
  spec_AFS_dm : FromWorkspace  VariableName=testSig_AFS_dm  Interpolate=off  OutputAfterFinalValue=Holding final value
  spec_AFS_dmDrft : FromWorkspace  VariableName=testSig_AFS_dmDrft  Interpolate=off  OutputAfterFinalValue=Holding final value
  spec_AFS_dmPlsCorr : FromWorkspace  VariableName=testSig_AFS_dmPlsCorr  Interpolate=off  OutputAfterFinalValue=Holding final value
  spec_AFS_dmSens : FromWorkspace  VariableName=testSig_AFS_dmSens  Interpolate=off  OutputAfterFinalValue=Holding final value
  spec_AFS_mAirPerCyl : FromWorkspace  VariableName=testSig_AFS_mAirPerCyl  Interpolate=off  OutputAfterFinalValue=Holding final value
  spec_AFS_stDrft : FromWorkspace  VariableName=testSig_AFS_stDrft  Interpolate=off  OutputAfterFinalValue=Holding final value
  spec_AFS_stDrftMonRls_mp : FromWorkspace  VariableName=testSig_AFS_stDrftMonRls_mp  Interpolate=off  OutputAfterFinalValue=Holding final value
  spec_ASMod_dmIndAirRef : FromWorkspace  VariableName=testSig_ASMod_dmIndAirRef  Interpolate=off  OutputAfterFinalValue=Holding final value
  spec_AirCtl_stMon : FromWorkspace  VariableName=testSig_AirCtl_stMon  Interpolate=off  OutputAfterFinalValue=Holding final value
  spec_Air_pIntkVUs : FromWorkspace  VariableName=testSig_Air_pIntkVUs  Interpolate=off  OutputAfterFinalValue=Holding final value
  spec_Air_tAFS_mp : FromWorkspace  VariableName=testSig_Air_tAFS_mp  Interpolate=off  OutputAfterFinalValue=Holding final value
  spec_Air_tIntkVUs : FromWorkspace  VariableName=testSig_Air_tIntkVUs  Interpolate=off  OutputAfterFinalValue=Holding final value
  spec_CEngDsT_t : FromWorkspace  VariableName=testSig_CEngDsT_t  Interpolate=off  OutputAfterFinalValue=Holding final value
  spec_CoEng_st : FromWorkspace  VariableName=testSig_CoEng_st  Interpolate=off  OutputAfterFinalValue=Holding final value
  spec_DSM_bAFS : FromWorkspace  VariableName=testSig_DSM_bAFS  Interpolate=off  OutputAfterFinalValue=Holding final value
  spec_DSM_bAFSActrTst : FromWorkspace  VariableName=testSig_DSM_bAFSActrTst  Interpolate=off  OutputAfterFinalValue=Holding final value
  spec_DSM_bAFSFrzAirMs : FromWorkspace  VariableName=testSig_DSM_bAFSFrzAirMs  Interpolate=off  OutputAfterFinalValue=Holding final value
  spec_DSM_bAFSPlSetyDrft : FromWorkspace  VariableName=testSig_DSM_bAFSPlSetyDrft  Interpolate=off  OutputAfterFinalValue=Holding final value
  spec_DSM_bAFSSysErr : FromWorkspace  VariableName=testSig_DSM_bAFSSysErr  Interpolate=off  OutputAfterFinalValue=Holding final value
  spec_EGRVlv_r : FromWorkspace  VariableName=testSig_EGRVlv_r  Interpolate=off  OutputAfterFinalValue=Holding final value
  spec_EngDa_tEng : FromWorkspace  VariableName=testSig_EngDa_tEng  Interpolate=off  OutputAfterFinalValue=Holding final value
  spec_EnvP_p : FromWorkspace  VariableName=testSig_EnvP_p  Interpolate=off  OutputAfterFinalValue=Holding final value
  spec_EnvT_t : FromWorkspace  VariableName=testSig_EnvT_t  Interpolate=off  OutputAfterFinalValue=Holding final value
  spec_Epm_nEng : FromWorkspace  VariableName=testSig_Epm_nEng  Interpolate=off  OutputAfterFinalValue=Holding final value
  spec_InjCtl_qRaw : FromWorkspace  VariableName=testSig_InjCtl_qRaw  Interpolate=off  OutputAfterFinalValue=Holding final value
  spec_InjCtl_qSetUnBal : FromWorkspace  VariableName=testSig_InjCtl_qSetUnBal  Interpolate=off  OutputAfterFinalValue=Holding final value
  spec_Oil_tSwmp : FromWorkspace  VariableName=testSig_Oil_tSwmp  Interpolate=off  OutputAfterFinalValue=Holding final value
  spec_ThrVlv_r : FromWorkspace  VariableName=testSig_ThrVlv_r  Interpolate=off  OutputAfterFinalValue=Holding final value
  testSignals : Outport
  wires:
  BC/1 -> testSignals/1
  spec_AFS_dmSens/1 -> BC/1  "testSig_AFS_dmSens"
  spec_Epm_nEng/1 -> BC/2  "testSig_Epm_nEng"
  spec_InjCtl_qSetUnBal/1 -> BC/3  "testSig_InjCtl_qSetUnBal"
  spec_AirCtl_stMon/1 -> BC/4  "testSig_AirCtl_stMon"
  spec_EnvP_p/1 -> BC/5  "testSig_EnvP_p"
  spec_CoEng_st/1 -> BC/6  "testSig_CoEng_st"
  spec_ThrVlv_r/1 -> BC/7  "testSig_ThrVlv_r"
  spec_EGRVlv_r/1 -> BC/8  "testSig_EGRVlv_r"
  spec_InjCtl_qRaw/1 -> BC/9  "testSig_InjCtl_qRaw"
  spec_Air_pIntkVUs/1 -> BC/10  "testSig_Air_pIntkVUs"
  spec_AFS_stDrft/1 -> BC/11  "testSig_AFS_stDrft"
  spec_ASMod_dmIndAirRef/1 -> BC/12  "testSig_ASMod_dmIndAirRef"
  spec_AFS_dmDrft/1 -> BC/13  "testSig_AFS_dmDrft"
  spec_DSM_bAFSFrzAirMs/1 -> BC/14  "testSig_DSM_bAFSFrzAirMs"
  spec_DSM_bAFSActrTst/1 -> BC/15  "testSig_DSM_bAFSActrTst"
  spec_DSM_bAFSPlSetyDrft/1 -> BC/16  "testSig_DSM_bAFSPlSetyDrft"
  spec_DSM_bAFSSysErr/1 -> BC/17  "testSig_DSM_bAFSSysErr"
  spec_DSM_bAFS/1 -> BC/18  "testSig_DSM_bAFS"
  spec_CEngDsT_t/1 -> BC/19  "testSig_CEngDsT_t"
  spec_Oil_tSwmp/1 -> BC/20  "testSig_Oil_tSwmp"
  spec_EngDa_tEng/1 -> BC/21  "testSig_EngDa_tEng"
  spec_Air_tAFS_mp/1 -> BC/22  "testSig_Air_tAFS_mp"
  spec_EnvT_t/1 -> BC/23  "testSig_EnvT_t"
  spec_Air_tIntkVUs/1 -> BC/24  "testSig_Air_tIntkVUs"
  spec_AFS_mAirPerCyl/1 -> BC/25  "testSig_AFS_mAirPerCyl"
  spec_AFS_dm/1 -> BC/26  "testSig_AFS_dm"
  spec_AFS_dmPlsCorr/1 -> BC/27  "testSig_AFS_dmPlsCorr"
  spec_AFS_stDrftMonRls_mp/1 -> BC/28  "testSig_AFS_stDrftMonRls_mp"
  spec_AFS_bPlausMinDeb_DSM/1 -> BC/29  "testSig_AFS_bPlausMinDeb_DSM"
  spec_AFS_bPlausMaxDeb_DSM/1 -> BC/30  "testSig_AFS_bPlausMaxDeb_DSM"

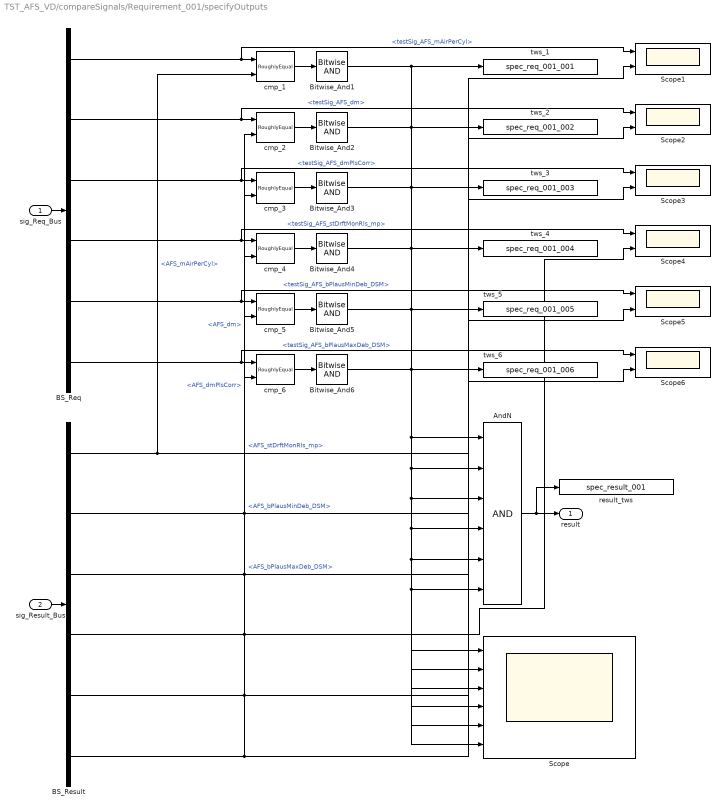
== system TST_AFS_VD/compareSignals/Requirement_001/specifyOutputs ==
  sig_Req_Bus : Inport
  sig_Result_Bus : Inport  Port=2
  AndN : Logic  Inputs=6
  BS_Req : BusSelector  OutputSignals=testSig_AFS_mAirPerCyl,testSig_AFS_dm,testSig_AFS_dmPlsCorr,testSig_AFS_stDrftMonRls_mp,testSig_AFS_bPlausMinDeb_DSM,testSig_AFS_bPlausMaxDeb_DSM
  BS_Result : BusSelector  OutputSignals=AFS_mAirPerCyl,AFS_dm,AFS_dmPlsCorr,AFS_stDrftMonRls_mp,AFS_bPlausMinDeb_DSM,AFS_bPlausMaxDeb_DSM
  Bitwise_And{1..6} (6 alike) : simulink/Logic and Bit Operations/Bitwise Operator  logicop=AND  UseBitMask=off  BitMask=bin2dec('11011001')  BitMaskRealWorld=Stored Integer
  Scope : Scope  NumInputPorts=6
  Scope{1..6} (6 alike) : Scope  NumInputPorts=2
  cmp_1 : UnitTest_Lib/RoughlyEqual  slope=10
  cmp_2 : UnitTest_Lib/RoughlyEqual  slope=2
  cmp_3 : UnitTest_Lib/RoughlyEqual  slope=2
  cmp_4 : UnitTest_Lib/RoughlyEqual  slope=0.1
  cmp_5 : UnitTest_Lib/RoughlyEqual  slope=0.1
  cmp_6 : UnitTest_Lib/RoughlyEqual  slope=0.1
  result_tws : ToWorkspace  VariableName=spec_result_001
  tws_1 : ToWorkspace  VariableName=spec_req_001_001
  tws_2 : ToWorkspace  VariableName=spec_req_001_002
  tws_3 : ToWorkspace  VariableName=spec_req_001_003
  tws_4 : ToWorkspace  VariableName=spec_req_001_004
  tws_5 : ToWorkspace  VariableName=spec_req_001_005
  tws_6 : ToWorkspace  VariableName=spec_req_001_006
  result : Outport
  wires:
  sig_Req_Bus/1 -> BS_Req/1
  sig_Result_Bus/1 -> BS_Result/1
  AndN/1 -> result/1, result_tws/1
  BS_Req/1 -> cmp_1/1, Scope1/1  "<testSig_AFS_mAirPerCyl>"
  BS_Result/1 -> cmp_1/2, Scope1/2  "<AFS_mAirPerCyl>"
  cmp_1/1 -> Bitwise_And1/1
  Bitwise_And1/1 -> AndN/1, Scope/1, tws_1/1
  BS_Req/2 -> cmp_2/1, Scope2/1  "<testSig_AFS_dm>"
  BS_Result/2 -> cmp_2/2, Scope2/2  "<AFS_dm>"
  cmp_2/1 -> Bitwise_And2/1
  Bitwise_And2/1 -> AndN/2, Scope/2, tws_2/1
  BS_Req/3 -> cmp_3/1, Scope3/1  "<testSig_AFS_dmPlsCorr>"
  BS_Result/3 -> cmp_3/2, Scope3/2  "<AFS_dmPlsCorr>"
  cmp_3/1 -> Bitwise_And3/1
  Bitwise_And3/1 -> AndN/3, Scope/3, tws_3/1
  BS_Req/4 -> cmp_4/1, Scope4/1  "<testSig_AFS_stDrftMonRls_mp>"
  BS_Result/4 -> cmp_4/2, Scope4/2  "<AFS_stDrftMonRls_mp>"
  cmp_4/1 -> Bitwise_And4/1
  Bitwise_And4/1 -> AndN/4, Scope/4, tws_4/1
  BS_Req/5 -> cmp_5/1, Scope5/1  "<testSig_AFS_bPlausMinDeb_DSM>"
  BS_Result/5 -> cmp_5/2, Scope5/2  "<AFS_bPlausMinDeb_DSM>"
  cmp_5/1 -> Bitwise_And5/1
  Bitwise_And5/1 -> AndN/5, Scope/5, tws_5/1
  BS_Req/6 -> cmp_6/1, Scope6/1  "<testSig_AFS_bPlausMaxDeb_DSM>"
  BS_Result/6 -> cmp_6/2, Scope6/2  "<AFS_bPlausMaxDeb_DSM>"
  cmp_6/1 -> Bitwise_And6/1
  Bitwise_And6/1 -> AndN/6, Scope/6, tws_6/1

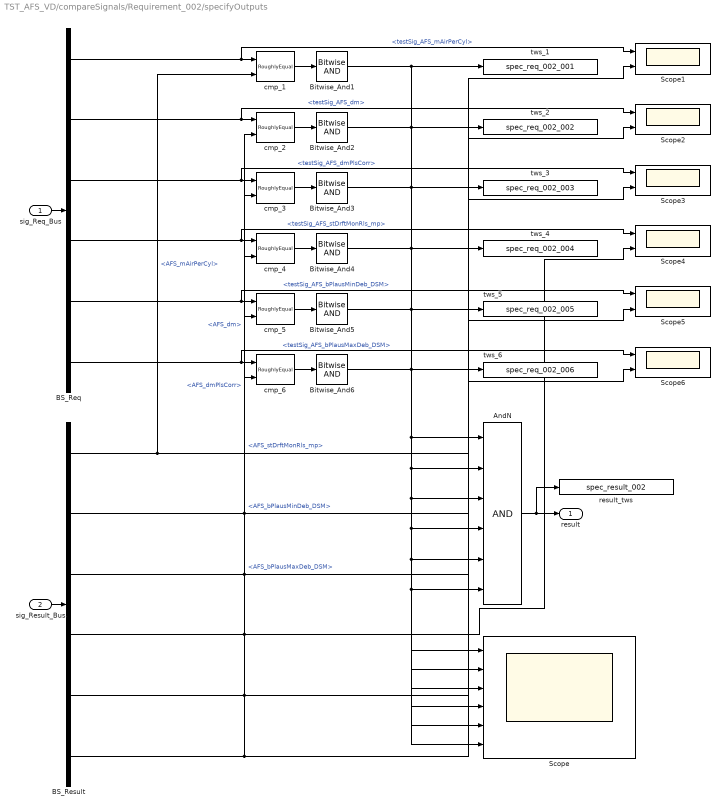
== system TST_AFS_VD/compareSignals/Requirement_002/specifyOutputs ==
  sig_Req_Bus : Inport
  sig_Result_Bus : Inport  Port=2
  AndN : Logic  Inputs=6
  BS_Req : BusSelector  OutputSignals=testSig_AFS_mAirPerCyl,testSig_AFS_dm,testSig_AFS_dmPlsCorr,testSig_AFS_stDrftMonRls_mp,testSig_AFS_bPlausMinDeb_DSM,testSig_AFS_bPlausMaxDeb_DSM
  BS_Result : BusSelector  OutputSignals=AFS_mAirPerCyl,AFS_dm,AFS_dmPlsCorr,AFS_stDrftMonRls_mp,AFS_bPlausMinDeb_DSM,AFS_bPlausMaxDeb_DSM
  Bitwise_And{1..6} (6 alike) : simulink/Logic and Bit Operations/Bitwise Operator  logicop=AND  UseBitMask=off  BitMask=bin2dec('11011001')  BitMaskRealWorld=Stored Integer
  Scope : Scope  NumInputPorts=6
  Scope{1..6} (6 alike) : Scope  NumInputPorts=2
  cmp_{1..2,4..6} (5 alike) : UnitTest_Lib/RoughlyEqual  slope=0.1
  cmp_3 : UnitTest_Lib/RoughlyEqual  slope=2
  result_tws : ToWorkspace  VariableName=spec_result_002
  tws_1 : ToWorkspace  VariableName=spec_req_002_001
  tws_2 : ToWorkspace  VariableName=spec_req_002_002
  tws_3 : ToWorkspace  VariableName=spec_req_002_003
  tws_4 : ToWorkspace  VariableName=spec_req_002_004
  tws_5 : ToWorkspace  VariableName=spec_req_002_005
  tws_6 : ToWorkspace  VariableName=spec_req_002_006
  result : Outport
  wires:
  sig_Req_Bus/1 -> BS_Req/1
  sig_Result_Bus/1 -> BS_Result/1
  AndN/1 -> result/1, result_tws/1
  BS_Req/1 -> cmp_1/1, Scope1/1  "<testSig_AFS_mAirPerCyl>"
  BS_Result/1 -> cmp_1/2, Scope1/2  "<AFS_mAirPerCyl>"
  cmp_1/1 -> Bitwise_And1/1
  Bitwise_And1/1 -> AndN/1, Scope/1, tws_1/1
  BS_Req/2 -> cmp_2/1, Scope2/1  "<testSig_AFS_dm>"
  BS_Result/2 -> cmp_2/2, Scope2/2  "<AFS_dm>"
  cmp_2/1 -> Bitwise_And2/1
  Bitwise_And2/1 -> AndN/2, Scope/2, tws_2/1
  BS_Req/3 -> cmp_3/1, Scope3/1  "<testSig_AFS_dmPlsCorr>"
  BS_Result/3 -> cmp_3/2, Scope3/2  "<AFS_dmPlsCorr>"
  cmp_3/1 -> Bitwise_And3/1
  Bitwise_And3/1 -> AndN/3, Scope/3, tws_3/1
  BS_Req/4 -> cmp_4/1, Scope4/1  "<testSig_AFS_stDrftMonRls_mp>"
  BS_Result/4 -> cmp_4/2, Scope4/2  "<AFS_stDrftMonRls_mp>"
  cmp_4/1 -> Bitwise_And4/1
  Bitwise_And4/1 -> AndN/4, Scope/4, tws_4/1
  BS_Req/5 -> cmp_5/1, Scope5/1  "<testSig_AFS_bPlausMinDeb_DSM>"
  BS_Result/5 -> cmp_5/2, Scope5/2  "<AFS_bPlausMinDeb_DSM>"
  cmp_5/1 -> Bitwise_And5/1
  Bitwise_And5/1 -> AndN/5, Scope/5, tws_5/1
  BS_Req/6 -> cmp_6/1, Scope6/1  "<testSig_AFS_bPlausMaxDeb_DSM>"
  BS_Result/6 -> cmp_6/2, Scope6/2  "<AFS_bPlausMaxDeb_DSM>"
  cmp_6/1 -> Bitwise_And6/1
  Bitwise_And6/1 -> AndN/6, Scope/6, tws_6/1
